simulink model "track_vehicle_simulation"  (R2018a)
settings: Solver=ode4  StartTime=0.0  StopTime=330  RelTol=1e-3
values from neighbouring files (symbols this model uses):
  coefficient_regarding_air = 0.0331    [initialize.m]
  desired_acceleration = 0.1 + desired_acceleration_samples_positions*0    [initialize.m]
  desired_acceleration_samples_positions = linspace(0, track_length-1, track_length)    [initialize.m]
  desired_speed = 7 + desired_speed_samples_positions*0    [initialize.m]
  desired_speed_samples_positions = linspace(0, track_length-1, track_length)    [initialize.m]
  desired_torque = 8 + desired_torque_samples_positions*0    [initialize.m]
  desired_torque_samples_positions = linspace(0, track_length-1, track_length)    [initialize.m]
  gravity_acceleration = 9.78    [initialize.m]
  interpolated_elevation = interpolated_elevation((extra_points_for_interpolation*interpolated_points_per_meter)+1:(track_length+extra_points_for_interpolation)*interpolated_points_per_meter)    [initialize.m]
  interpolated_positions = linspace(0,track_length, track_length*interpolated_points_per_meter)    [initialize.m]
  interpolated_slope = interpolated_slope((extra_points_for_interpolation*interpolated_points_per_meter)+1:(track_length+extra_points_for_interpolation)*interpolated_points_per_meter)    [initialize.m]
  ki = 0.01    [initialize.m]
  kp = 3    [initialize.m]
  max_torque = 15    [initialize.m]
  min_torque = 0    [initialize.m]
  rolling_resistance_factor = 0.0024    [initialize.m]
  track_length = 2244    [from_excel_to_mat.m]    (also in track_data.mat)
  Ts = 1e-3    (= 0.001)    [initialize.m]
  vehicle_mass = 90    [initialize.m]
  wheel_radius = 0.239    [initialize.m]
undefined symbols (not defined in the file or in its folder): DiscIntNeverNeededParam
libraries: dspstat3 x3, simulink x1
settings Model: Creator=el16077  LastModifiedBy=el16077

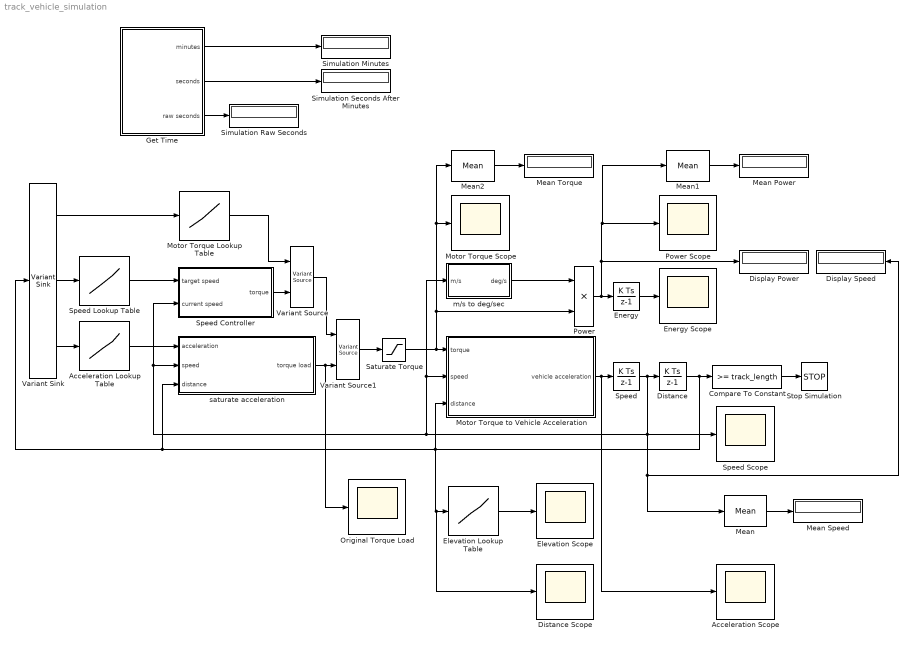
== system track_vehicle_simulation ==
  Acceleration Lookup Table : Lookup_n-D  NumberOfTableDimensions=1  BreakpointsForDimension1=desired_acceleration_samples_positions  Table=desired_acceleration  InternalRulePriority=Speed  RndMeth=Simplest  InputSameDT=on
  Acceleration Scope : Scope
  Compare To Constant : simulink/Logic and Bit Operations/Compare To Constant  relop=>=  const=track_length  OutDataTypeStr=boolean
  Display Power : Display
  Display Speed : Display
  Distance : DiscreteIntegrator  SampleTime=Ts  ICPrevOutput=DiscIntNeverNeededParam  ICPrevScaledInput=DiscIntNeverNeededParam
  Distance Scope : Scope
  Elevation Lookup Table : Lookup_n-D  NumberOfTableDimensions=1  BreakpointsForDimension1=interpolated_positions  Table=interpolated_elevation  InternalRulePriority=Speed  RndMeth=Simplest  InputSameDT=on
  Elevation Scope : Scope
  Energy : DiscreteIntegrator  gainval=0.1  SampleTime=Ts  ICPrevOutput=DiscIntNeverNeededParam  ICPrevScaledInput=DiscIntNeverNeededParam
  Energy Scope : Scope
  Get Time : Subsystem
  Mean : dspstat3/Mean  run=on  reset_popup=None  directionMode=Each column  dimension=1  roiEnable=off  roiType=Rectangles  roiPortion=Entire ROI  roiOutput=Individual statistics for each ROI  roiFlag=off  roundingMode=Floor  overflowMode=off  outputDataTypeStr=Inherit: Same as accumulator  outputMin=[]  outputMax=[]  outputLastDataTypeStr=Inherit: Same as accumulator
  Mean Power : Display
  Mean Speed : Display
  Mean Torque : Display
  Mean1 : dspstat3/Mean  run=on  reset_popup=None  directionMode=Each column  dimension=1  roiEnable=off  roiType=Rectangles  roiPortion=Entire ROI  roiOutput=Individual statistics for each ROI  roiFlag=off  roundingMode=Floor  overflowMode=off  outputDataTypeStr=Inherit: Same as accumulator  outputMin=[]  outputMax=[]  outputLastDataTypeStr=Inherit: Same as accumulator
  Mean2 : dspstat3/Mean  run=on  reset_popup=None  directionMode=Each column  dimension=1  roiEnable=off  roiType=Rectangles  roiPortion=Entire ROI  roiOutput=Individual statistics for each ROI  roiFlag=off  roundingMode=Floor  overflowMode=off  outputDataTypeStr=Inherit: Same as accumulator  outputMin=[]  outputMax=[]  outputLastDataTypeStr=Inherit: Same as accumulator
  Motor Torque Lookup Table : Lookup_n-D  NumberOfTableDimensions=1  BreakpointsForDimension1=desired_torque_samples_positions  Table=desired_torque  InternalRulePriority=Speed  RndMeth=Simplest  InputSameDT=on
  Motor Torque Scope : Scope
  Motor Torque to Vehicle Acceleration : Subsystem
  Original Torque Load : Scope
  Power : Product
  Power Scope : Scope
  Saturate Torque : Saturate  UpperLimit=max_torque  LowerLimit=min_torque
  Simulation Minutes : Display
  Simulation Raw Seconds : Display
  Simulation Seconds After Minutes : Display
  Speed : DiscreteIntegrator  SampleTime=Ts  ICPrevOutput=DiscIntNeverNeededParam  ICPrevScaledInput=DiscIntNeverNeededParam
  Speed Controller : Subsystem
  Speed Lookup Table : Lookup_n-D  NumberOfTableDimensions=1  BreakpointsForDimension1=desired_speed_samples_positions  Table=desired_speed  InternalRulePriority=Speed  RndMeth=Simplest  InputSameDT=on
  Speed Scope : Scope
  Stop Simulation : Stop
  Variant Sink : VariantSink
  Variant Source : VariantSource
      settings: AllowZeroVariantControls=on
  Variant Source1 : VariantSource
  m/s to deg/sec : Subsystem
  saturate acceleration : Subsystem
  wires:
  Get Time/1(minutes) -> Simulation Minutes/1
  Get Time/2(seconds) -> Simulation Seconds After Minutes/1
  Get Time/3(raw seconds) -> Simulation Raw Seconds/1
  Motor Torque to Vehicle Acceleration/1(vehicle acceleration) -> Acceleration Scope/1, Speed/1
  Speed/1 -> Mean/1, Display Speed/1, Speed Scope/1, Speed Controller/2(current speed), saturate acceleration/2(speed), m/s to deg/sec/1(m/s), Motor Torque to Vehicle Acceleration/2(speed), Distance/1
  m/s to deg/sec/1(deg/s) -> Power/1
  Power/1 -> Mean1/1, Power Scope/1, Display Power/1, Energy/1
  Saturate Torque/1 -> Mean2/1, Motor Torque Scope/1, Power/2, Motor Torque to Vehicle Acceleration/1(torque)
  Distance/1 -> Variant Sink/1, saturate acceleration/3(distance), Motor Torque to Vehicle Acceleration/3(distance), Distance Scope/1, Elevation Lookup Table/1, Compare To Constant/1
  Compare To Constant/1 -> Stop Simulation/1
  Energy/1 -> Energy Scope/1
  Elevation Lookup Table/1 -> Elevation Scope/1
  Variant Source1/1 -> Saturate Torque/1
  Acceleration Lookup Table/1 -> saturate acceleration/1(acceleration)
  Motor Torque Lookup Table/1 -> Variant Source/1
  Speed Lookup Table/1 -> Speed Controller/1(target speed)
  Speed Controller/1(torque) -> Variant Source/2
  Variant Source/1 -> Variant Source1/1
  Variant Sink/3 -> Acceleration Lookup Table/1
  Variant Sink/2 -> Speed Lookup Table/1
  Variant Sink/1 -> Motor Torque Lookup Table/1
  saturate acceleration/1(torque load) -> Original Torque Load/1, Variant Source1/2
  Mean/1 -> Mean Speed/1
  Mean1/1 -> Mean Power/1
  Mean2/1 -> Mean Torque/1

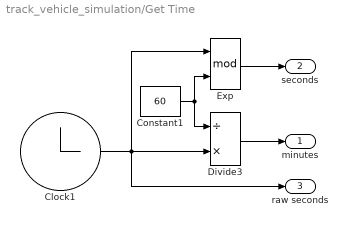
== system track_vehicle_simulation/Get Time ==
  Clock1 : Clock
      settings: Decimation=1/Ts
  Constant1 : Constant  Value=60
  Divide3 : Product  Inputs=/*  OutDataTypeStr=fixdt('int8', 'DataTypeOverride', 'Off')
  Exp : Math  Operator=mod  SaturateOnIntegerOverflow=on
  minutes : Outport
  seconds : Outport  Port=2
  raw seconds : Outport  Port=3
  wires:
  Clock1/1 -> raw seconds/1, Exp/1, Divide3/2
  Constant1/1 -> Exp/2, Divide3/1
  Exp/1 -> seconds/1
  Divide3/1 -> minutes/1

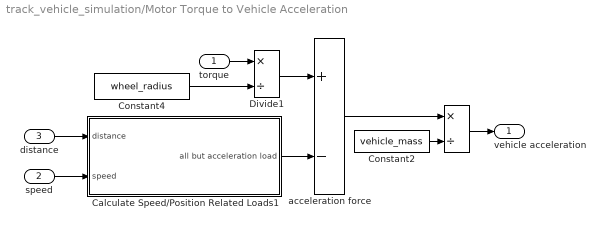
== system track_vehicle_simulation/Motor Torque to Vehicle Acceleration ==
  torque : Inport
  speed : Inport  Port=2
  distance : Inport  Port=3
  " " : Product  Inputs=*/
  Calculate Speed/Position Related Loads1 : Subsystem
  Constant2 : Constant  Value=vehicle_mass  SampleTime=Ts
  Constant4 : Constant  Value=wheel_radius  SampleTime=Ts
  Divide1 : Product  Inputs=*/
  acceleration force : Sum  Inputs=+-
  vehicle acceleration : Outport
  wires:
  " "/1 -> vehicle acceleration/1
  distance/1 -> Calculate Speed/Position Related Loads1/1(distance)
  Divide1/1 -> acceleration force/1
  acceleration force/1 -> " "/1
  torque/1 -> Divide1/1
  speed/1 -> Calculate Speed/Position Related Loads1/2(speed)
  Calculate Speed/Position Related Loads1/1(all but acceleration load) -> acceleration force/2
  Constant4/1 -> Divide1/2
  Constant2/1 -> " "/2

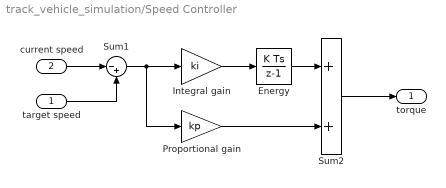
== system track_vehicle_simulation/Speed Controller ==
  target speed : Inport
  current speed : Inport  Port=2
  Energy : DiscreteIntegrator  gainval=0.1  SampleTime=Ts  ICPrevOutput=DiscIntNeverNeededParam  ICPrevScaledInput=DiscIntNeverNeededParam
  Integral gain : Gain  Gain=ki  SaturateOnIntegerOverflow=on  OutDataTypeStr=Inherit: Same as input  ParamDataTypeStr=Inherit: Same as input
  Proportional gain : Gain  Gain=kp  SaturateOnIntegerOverflow=on  OutDataTypeStr=Inherit: Same as input  ParamDataTypeStr=Inherit: Same as input
  Sum1 : Sum  Inputs=|-+  SaturateOnIntegerOverflow=on  InputSameDT=on  OutDataTypeStr=Inherit: Same as first input
  Sum2 : Sum  SaturateOnIntegerOverflow=on  InputSameDT=on  OutDataTypeStr=Inherit: Same as first input
  torque : Outport
  wires:
  current speed/1 -> Sum1/1
  target speed/1 -> Sum1/2
  Sum2/1 -> torque/1
  Proportional gain/1 -> Sum2/2
  Energy/1 -> Sum2/1
  Sum1/1 -> Proportional gain/1, Integral gain/1
  Integral gain/1 -> Energy/1

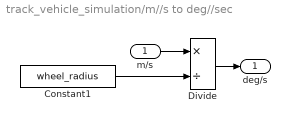
== system track_vehicle_simulation/m//s to deg//sec ==
  m/s : Inport
  Constant1 : Constant  Value=wheel_radius  SampleTime=Ts
  Divide : Product  Inputs=*/
  deg/s : Outport
  wires:
  Constant1/1 -> Divide/2
  m/s/1 -> Divide/1
  Divide/1 -> deg/s/1

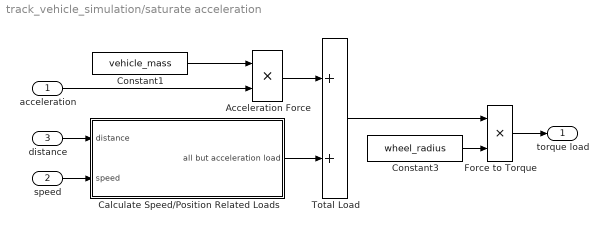
== system track_vehicle_simulation/saturate acceleration ==
  acceleration : Inport
  speed : Inport  Port=2
  distance : Inport  Port=3
  Acceleration Force : Product  SampleTime=Ts
  Calculate Speed/Position Related Loads : Subsystem
  Constant1 : Constant  Value=vehicle_mass  SampleTime=Ts
  Constant3 : Constant  Value=wheel_radius  SampleTime=Ts
  Force to Torque : Product  SampleTime=Ts
  Total Load : Sum
  torque load : Outport
  wires:
  speed/1 -> Calculate Speed/Position Related Loads/2(speed)
  distance/1 -> Calculate Speed/Position Related Loads/1(distance)
  acceleration/1 -> Acceleration Force/2
  Constant1/1 -> Acceleration Force/1
  Total Load/1 -> Force to Torque/1
  Force to Torque/1 -> torque load/1
  Constant3/1 -> Force to Torque/2
  Acceleration Force/1 -> Total Load/1
  Calculate Speed/Position Related Loads/1(all but acceleration load) -> Total Load/2

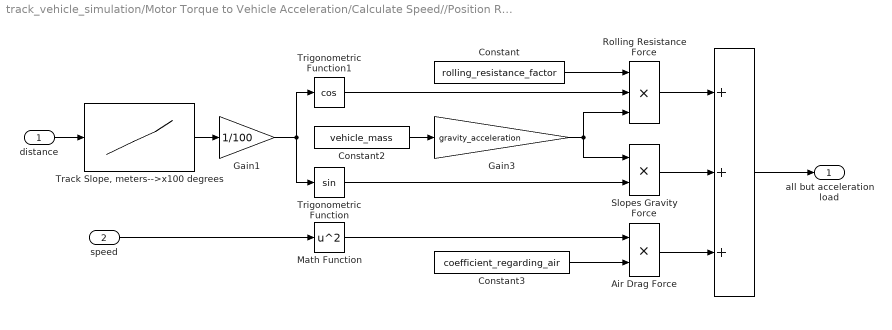
== system track_vehicle_simulation/Motor Torque to Vehicle Acceleration/Calculate Speed//Position Related Loads1 ==
  distance : Inport
  speed : Inport  Port=2
  " " : Sum  Inputs=+++
  Air Drag Force : Product  SampleTime=Ts
  Constant : Constant  Value=rolling_resistance_factor  SampleTime=Ts
  Constant2 : Constant  Value=vehicle_mass  SampleTime=Ts
  Constant3 : Constant  Value=coefficient_regarding_air  SampleTime=Ts
  Gain1 : Gain  Gain=1/100  SampleTime=Ts
  Gain3 : Gain  Gain=gravity_acceleration  SampleTime=Ts
  Math Function : Math  Operator=square  SaturateOnIntegerOverflow=on
  Rolling Resistance Force : Product  Inputs=3  SampleTime=Ts
  Slopes Gravity Force : Product  SampleTime=Ts
  "Track Slope, meters-->x100 degrees" : Lookup_n-D  NumberOfTableDimensions=1  BreakpointsForDimension1=interpolated_positions  Table=interpolated_slope  InternalRulePriority=Speed  RndMeth=Simplest  InputSameDT=on
  Trigonometric Function : Trigonometry  SampleTime=Ts
  Trigonometric Function1 : Trigonometry  Operator=cos  SampleTime=Ts
  all but acceleration load : Outport
  wires:
  " "/1 -> all but acceleration load/1
  Constant3/1 -> Air Drag Force/2
  Constant/1 -> Rolling Resistance Force/1
  Gain1/1 -> Trigonometric Function/1, Trigonometric Function1/1
  Trigonometric Function/1 -> Slopes Gravity Force/2
  Gain3/1 -> Rolling Resistance Force/3, Slopes Gravity Force/1
  Trigonometric Function1/1 -> Rolling Resistance Force/2
  Constant2/1 -> Gain3/1
  Math Function/1 -> Air Drag Force/1
  speed/1 -> Math Function/1
  Air Drag Force/1 -> " "/3
  Slopes Gravity Force/1 -> " "/2
  Rolling Resistance Force/1 -> " "/1
  distance/1 -> "Track Slope, meters-->x100 degrees"/1
  "Track Slope, meters-->x100 degrees"/1 -> Gain1/1

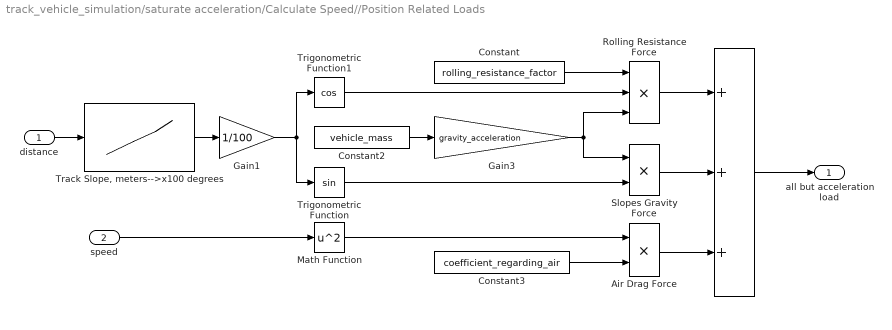
== system track_vehicle_simulation/saturate acceleration/Calculate Speed//Position Related Loads ==
  distance : Inport
  speed : Inport  Port=2
  " " : Sum  Inputs=+++
  Air Drag Force : Product  SampleTime=Ts
  Constant : Constant  Value=rolling_resistance_factor  SampleTime=Ts
  Constant2 : Constant  Value=vehicle_mass  SampleTime=Ts
  Constant3 : Constant  Value=coefficient_regarding_air  SampleTime=Ts
  Gain1 : Gain  Gain=1/100  SampleTime=Ts
  Gain3 : Gain  Gain=gravity_acceleration  SampleTime=Ts
  Math Function : Math  Operator=square  SaturateOnIntegerOverflow=on
  Rolling Resistance Force : Product  Inputs=3  SampleTime=Ts
  Slopes Gravity Force : Product  SampleTime=Ts
  "Track Slope, meters-->x100 degrees" : Lookup_n-D  NumberOfTableDimensions=1  BreakpointsForDimension1=interpolated_positions  Table=interpolated_slope  InternalRulePriority=Speed  RndMeth=Simplest  InputSameDT=on
  Trigonometric Function : Trigonometry  SampleTime=Ts
  Trigonometric Function1 : Trigonometry  Operator=cos  SampleTime=Ts
  all but acceleration load : Outport
  wires:
  " "/1 -> all but acceleration load/1
  Constant3/1 -> Air Drag Force/2
  Constant/1 -> Rolling Resistance Force/1
  Gain1/1 -> Trigonometric Function/1, Trigonometric Function1/1
  Trigonometric Function/1 -> Slopes Gravity Force/2
  Gain3/1 -> Rolling Resistance Force/3, Slopes Gravity Force/1
  Trigonometric Function1/1 -> Rolling Resistance Force/2
  Constant2/1 -> Gain3/1
  Math Function/1 -> Air Drag Force/1
  speed/1 -> Math Function/1
  Air Drag Force/1 -> " "/3
  Slopes Gravity Force/1 -> " "/2
  Rolling Resistance Force/1 -> " "/1
  distance/1 -> "Track Slope, meters-->x100 degrees"/1
  "Track Slope, meters-->x100 degrees"/1 -> Gain1/1
